simulink model "DC_Motor"  (R2021a)
settings: Solver=VariableStepAuto  StartTime=0.0  StopTime=10.0  RelTol=1e-3
settings Model: Creator=serkan  LastModifiedBy=serkan

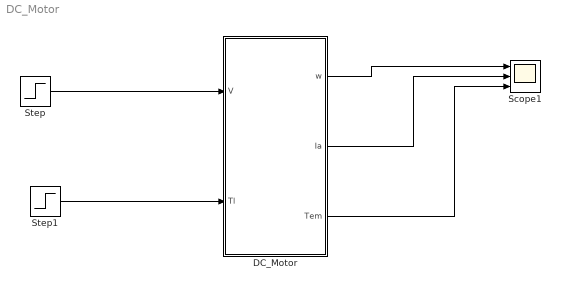
== system DC_Motor ==
  DC_Motor : Subsystem  mask{L=0.1, kt=0.5, Ra=0.45, J=0.1, b=0.2}
  Scope1 : Scope  NumInputPorts=3
  Step : Step  Time=0  After=25
  Step1 : Step  Time=2  After=10
  wires:
  Step/1 -> DC_Motor/1(V)
  Step1/1 -> DC_Motor/2(Tl)
  DC_Motor/3(Tem) -> Scope1/3
  DC_Motor/2(Ia) -> Scope1/2
  DC_Motor/1(w) -> Scope1/1

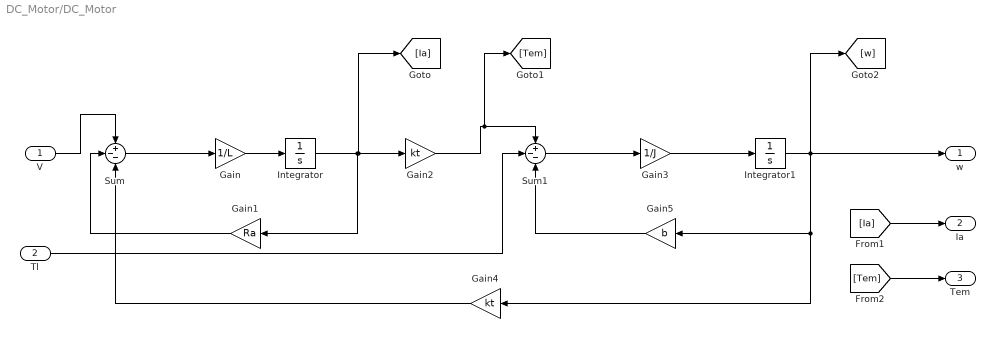
== system DC_Motor/DC_Motor ==
  V : Inport
  Tl : Inport  Port=2
  Gain : Gain  Gain=1/L
  Gain1 : Gain  Gain=Ra
  Gain2 : Gain  Gain=kt
  Gain3 : Gain  Gain=1/J
  Gain4 : Gain  Gain=kt
  Gain5 : Gain  Gain=b
  Integrator : Integrator
  Integrator1 : Integrator
  Sum : Sum  Inputs=+--
  Sum1 : Sum  Inputs=+--
  w : Outport
  Ia : Outport  Port=2
  Tem : Outport  Port=3
  wires:
  V/1 -> Sum/1
  Sum/1 -> Gain/1
  Gain/1 -> Integrator/1
  Integrator/1 -> Gain2/1, [Ia], Gain1/1
  Gain1/1 -> Sum/2
  Gain2/1 -> [Tem], Sum1/1
  Tl/1 -> Sum1/2
  Sum1/1 -> Gain3/1
  Gain3/1 -> Integrator1/1
  Integrator1/1 -> [w], Gain5/1, Gain4/1, w/1
  [Ia] -> Ia/1
  [Tem] -> Tem/1
  Gain4/1 -> Sum/3
  Gain5/1 -> Sum1/3
